simulink model "ask21"  (R2016a)
settings: Solver=VariableStepAuto  StartTime=0.0  StopTime=10.0  RelTol=1e-3
values from neighbouring files (symbols this model uses):
  A = [0 1 0 0;20.6 0 0 0;0 0 0 1;-0.5 0 0 0]    [ex2.m]
  B = [0;-1;0;0.5]    [ex2.m]
  initial = [-0.2;-0.06;0.01;0.3]    [ex2.m]
  K1 = (ad-a0)*T    [ex2.m]
settings Model: Creator=JIM  LastModifiedBy=JIM

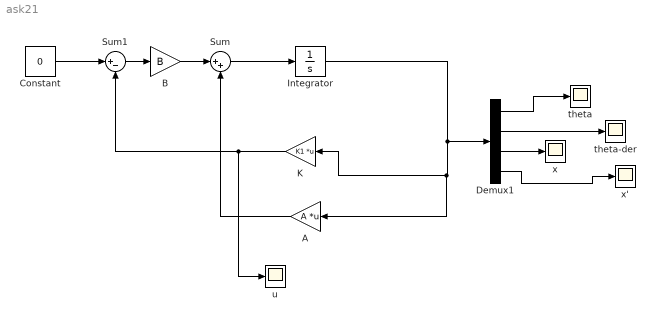
== system ask21 ==
  A : Gain  Gain=A  Multiplication=Matrix(K*u)
  B : Gain  Gain=B
  Constant : Constant  Value=0
  Demux1 : Demux
  Integrator : Integrator  InitialCondition=initial
  K : Gain  Gain=K1  Multiplication=Matrix(K*u)
  Sum : Sum  Inputs=|++
  Sum1 : Sum  Inputs=|+-
  theta : Scope
  theta-der : Scope
  u : Scope
  x : Scope
  "x' " : Scope
  wires:
  A/1 -> Sum/2
  Sum/1 -> Integrator/1
  K/1 -> Sum1/2, u/1
  Constant/1 -> Sum1/1
  Sum1/1 -> B/1
  B/1 -> Sum/1
  Integrator/1 -> A/1, K/1, Demux1/1
  Demux1/1 -> theta/1
  Demux1/2 -> theta-der/1
  Demux1/3 -> x/1
  Demux1/4 -> "x' "/1
